simulink model "robot"  (R2020a)
settings: Solver=VariableStepAuto  StartTime=0.0  StopTime=10  RelTol=1e-3
values from neighbouring files (symbols this model uses):
  den1 = [1 b*(i+m*l^2)/q1 -(M+m)*m*g*l/q1 -b*m*g*l/q1]    [params.m]
  num1 = [m*l/q1 0]    [params.m]
undefined symbols (not defined in the file or in its folder): DiscIntNeverNeededParam, Ts
libraries: simulink x2, rllib x1
settings Model: Creator=Preload  LastModifiedBy=User
settings DataIOCC: ReturnWorkspaceOutputs=off
settings DebuggingCC: ArithmeticOperatorsInVariantConditions=warning
settings SFSimCC: SimUseLocalCustomCode=off  CustomCodeUndefinedFunction=UseInterfaceOnly
settings RTWCC: RTWUseLocalCustomCode=off

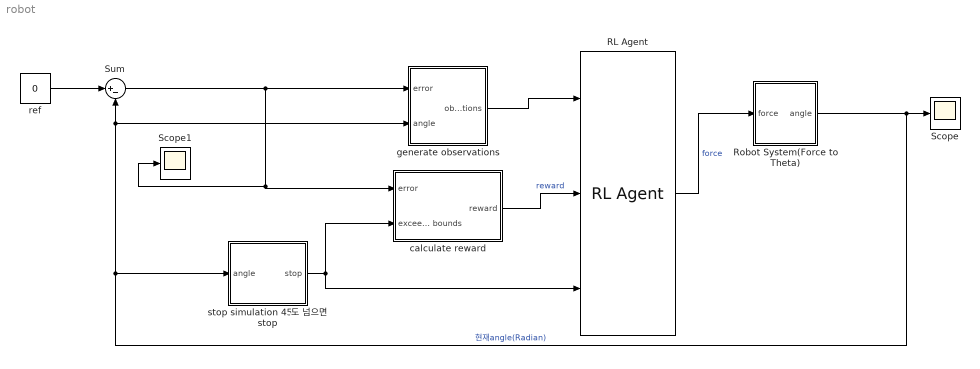
== system robot ==
  RL Agent : rllib/RL Agent  Agent=agent  ProvideReward=on  ProvideIsDone=on  ProvideCumRwd=off  TreatAsDirectFeedthrough=on  CollectLoggedSignals=on  CollectModelStates=on
  Robot System(Force to Theta) : Subsystem
  Scope : Scope
  Scope1 : Scope
  Sum : Sum  Inputs=|+-
  calculate reward : Subsystem
  generate observations : Subsystem
  ref : Constant  Value=0
  stop simulation 45도 넘으면 stop : Subsystem
  wires:
  ref/1 -> Sum/1
  RL Agent/1 -> Robot System(Force to Theta)/1(force)  "force"
  stop simulation 45도 넘으면 stop/1(stop) -> RL Agent/3, calculate reward/2(exceeds bounds)
  calculate reward/1(reward) -> RL Agent/2  "reward"
  Sum/1 -> Scope1/1, calculate reward/1(error), generate observations/1(error)
  Robot System(Force to Theta)/1(angle) -> Scope/1, stop simulation 45도 넘으면 stop/1(angle), Sum/2, generate observations/2(angle)  "현재angle(Radian)"
  generate observations/1(observations) -> RL Agent/1

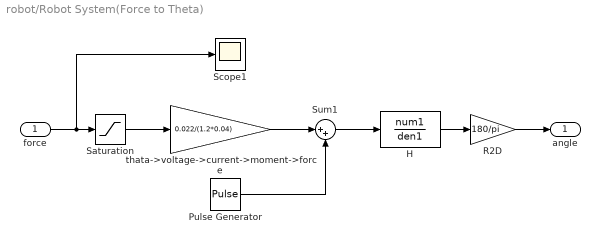
== system robot/Robot System(Force to Theta) ==
  force : Inport
  H : TransferFcn  Numerator=num1  Denominator=den1
  Pulse Generator : DiscretePulseGenerator  PulseType=Time based  Period=10  PulseWidth=0.1  PhaseDelay=0.1
  R2D : Gain  Gain=180/pi
  Saturation : Saturate  UpperLimit=12  LowerLimit=-12
  Scope1 : Scope
  Sum1 : Sum  Inputs=|++
  thata->voltage->current->moment->force : Gain  Gain=0.022/(1.2*0.04)
  angle : Outport
  wires:
  force/1 -> Scope1/1, Saturation/1
  Saturation/1 -> thata->voltage->current->moment->force/1
  Pulse Generator/1 -> Sum1/2
  thata->voltage->current->moment->force/1 -> Sum1/1
  H/1 -> R2D/1
  Sum1/1 -> H/1
  R2D/1 -> angle/1

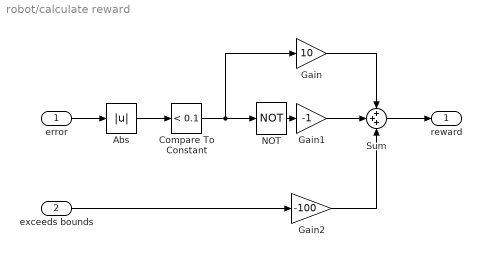
== system robot/calculate reward ==
  error : Inport
  exceeds bounds : Inport  Port=2
  Abs : Abs
  Compare To Constant : simulink/Logic and Bit Operations/Compare To Constant  relop=<  const=0.1  OutDataTypeStr=boolean
  Gain : Gain  Gain=10
  Gain1 : Gain  Gain=-1
  Gain2 : Gain  Gain=-100
  NOT : Logic  Operator=NOT  IconShape=distinctive  AllPortsSameDT=off  OutDataTypeStr=boolean
  Sum : Sum  Inputs=+++  OutDataTypeStr=double
  reward : Outport  VectorParamsAs1DForOutWhenUnconnected=off
  wires:
  Abs/1 -> Compare To Constant/1
  Gain2/1 -> Sum/3
  Gain/1 -> Sum/1
  Compare To Constant/1 -> NOT/1, Gain/1
  Gain1/1 -> Sum/2
  Sum/1 -> reward/1
  NOT/1 -> Gain1/1
  exceeds bounds/1 -> Gain2/1
  error/1 -> Abs/1

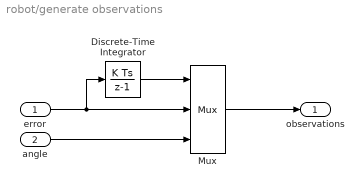
== system robot/generate observations ==
  error : Inport
  angle : Inport  Port=2
  Discrete-Time Integrator : DiscreteIntegrator  SampleTime=Ts  ICPrevOutput=DiscIntNeverNeededParam  ICPrevScaledInput=DiscIntNeverNeededParam
  Mux : Mux  Inputs=3
  observations : Outport  VectorParamsAs1DForOutWhenUnconnected=off
  wires:
  angle/1 -> Mux/3
  Discrete-Time Integrator/1 -> Mux/1
  error/1 -> Discrete-Time Integrator/1, Mux/2
  Mux/1 -> observations/1

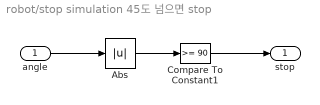
== system robot/stop simulation 45도 넘으면 stop ==
  angle : Inport
  Abs : Abs
  Compare To Constant1 : simulink/Logic and Bit Operations/Compare To Constant  relop=>=  const=90  OutDataTypeStr=boolean
  stop : Outport  VectorParamsAs1DForOutWhenUnconnected=off
  wires:
  Compare To Constant1/1 -> stop/1
  Abs/1 -> Compare To Constant1/1
  angle/1 -> Abs/1
